simulink model "Lab_06_Task03"  (R2015a)
settings: Solver=ode45  StartTime=0.0  StopTime=10.0  RelTol=1e-3
settings Model: Creator=Amir  LastModifiedBy=Amir

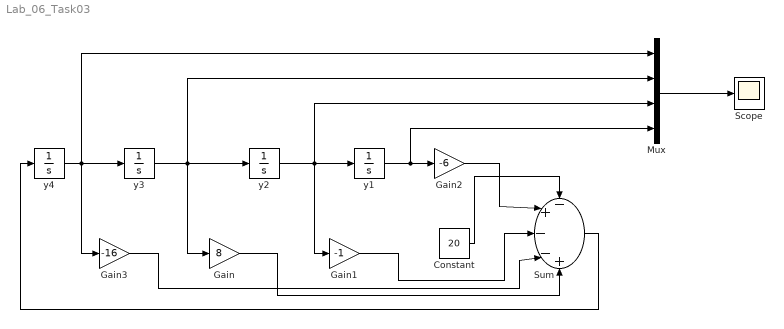
== system Lab_06_Task03 ==
  Constant : Constant  Value=20
  Gain : Gain  Gain=8
  Gain1 : Gain  Gain=-1
  Gain2 : Gain  Gain=-6
  Gain3 : Gain  Gain=-16
  Mux : Mux
  Scope : Scope
  Sum : Sum  Inputs=-+--+
  y1 : Integrator  InitialCondition=3
  y2 : Integrator  InitialCondition=10
  y3 : Integrator  InitialCondition=-6
  y4 : Integrator  InitialCondition=8
  wires:
  y1/1 -> Mux/4, Gain2/1
  y2/1 -> Mux/3, Gain1/1, y1/1
  y3/1 -> Mux/2, Gain/1, y2/1
  y4/1 -> Mux/1, Gain3/1, y3/1
  Gain2/1 -> Sum/2
  Constant/1 -> Sum/1
  Gain1/1 -> Sum/3
  Gain/1 -> Sum/5
  Gain3/1 -> Sum/4
  Mux/1 -> Scope/1
  Sum/1 -> y4/1
